simulink model "PandID"  (R2019b)
settings: Solver=VariableStepAuto  StartTime=0.0  StopTime=50  RelTol=1e-3
values from neighbouring files (symbols this model uses):
  L_area = 1    [AFCP_sim.m]
  P_area = 1    [AFCP_sim.m]
  PressureUnit = 1/6894.76    (= 0.000145037680789)    [AFCP_sim.m]
  R_area = 1    [AFCP_sim.m]
  Valve_signal_Unit = 0.00064516    [AFCP_sim.m]
libraries: fl_lib x96, nesl_utility x62, SimscapeFluids_lib x15, simulink x4
(part 2 of 2)

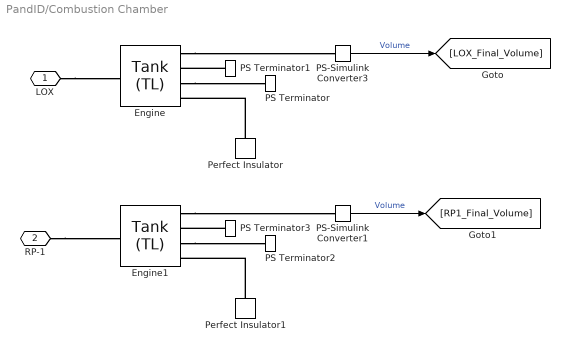
== system PandID/Combustion Chamber ==
  Engine : SimscapeFluids_lib/Thermal Liquid/Tanks & Accumulators/Tank (TL)  pressure_spec=1  tank_pressure=0.101325 MPa  max_capacity=100 m^3  volume_spec=1  tank_area=3 m^2  level_TLU=[0, 3, 5] m  volume_TLU=[0, 4, 6] m^3  inlet_height=0.1 m  inlet_area=0.01 m^2  g=9.81 m/s^2  level_specify=off  level_priority=Low  level=5 m  level_nominal_specify=off  level_nominal_unit=m  level_nominal_value=1  volume_specify=off  volume_priority=Low  volume=5 m^3  volume_nominal_specify=off  volume_nominal_unit=m^3  volume_nominal_value=1  mass_specify=off  mass_priority=Low  mass=5e+3 kg  mass_nominal_specify=off  mass_nominal_unit=kg  mass_nominal_value=1  T_tank_specify=off  T_tank_priority=Low  T_tank=293.15 K  T_tank_nominal_specify=off  T_tank_nominal_unit=K  T_tank_nominal_value=1  inlet_heights_AB=[.1, 0] m  inlet_areas_AB=[L_area, R_area] in^2  inlet_heights_ABC=[.1, .05, 0] m  inlet_areas_ABC=[.01, .01, .01] m^2
      settings: SourceProductName=Simscape Fluids  SourceProductBaseCode=SH  InternalSimscapePortConfiguration="{\"Bottom\":[],\"Left\":[{\"id\":\"A\",\"label\":\"A\",\"type\":\"foundation.thermal_liquid.thermal_liquid\"}],\"Right\":[{\"id\":\"V_out\",\"label\":\"V\",\"type\":\"output\"},{\"id\":\"L_out\",\"label\":\"L\",\"type\":\"output\"},{\"id\":\"T_out\",\"label\":\"T\",\"type\":\"output\"},{\"id\":\"H\",\"label\":\"H\",\"type\":\"foundation.thermal.thermal\"}],\"Top\":[]}"
  Engine1 : SimscapeFluids_lib/Thermal Liquid/Tanks & Accumulators/Tank (TL)  pressure_spec=1  tank_pressure=0.101325 MPa  max_capacity=100 m^3  volume_spec=1  tank_area=3 m^2  level_TLU=[0, 3, 5] m  volume_TLU=[0, 4, 6] m^3  inlet_height=0.1 m  inlet_area=0.01 m^2  g=9.81 m/s^2  level_specify=off  level_priority=Low  level=5 m  level_nominal_specify=off  level_nominal_unit=m  level_nominal_value=1  volume_specify=off  volume_priority=Low  volume=5 m^3  volume_nominal_specify=off  volume_nominal_unit=m^3  volume_nominal_value=1  mass_specify=off  mass_priority=Low  mass=5e+3 kg  mass_nominal_specify=off  mass_nominal_unit=kg  mass_nominal_value=1  T_tank_specify=off  T_tank_priority=Low  T_tank=293.15 K  T_tank_nominal_specify=off  T_tank_nominal_unit=K  T_tank_nominal_value=1  inlet_heights_AB=[.1, 0] m  inlet_areas_AB=[L_area, R_area] in^2  inlet_heights_ABC=[.1, .05, 0] m  inlet_areas_ABC=[.01, .01, .01] m^2
      settings: SourceProductName=Simscape Fluids  SourceProductBaseCode=SH  InternalSimscapePortConfiguration="{\"Bottom\":[],\"Left\":[{\"id\":\"A\",\"label\":\"A\",\"type\":\"foundation.thermal_liquid.thermal_liquid\"}],\"Right\":[{\"id\":\"V_out\",\"label\":\"V\",\"type\":\"output\"},{\"id\":\"L_out\",\"label\":\"L\",\"type\":\"output\"},{\"id\":\"T_out\",\"label\":\"T\",\"type\":\"output\"},{\"id\":\"H\",\"label\":\"H\",\"type\":\"foundation.thermal.thermal\"}],\"Top\":[]}"
  PS Terminator{,1..3} (4 alike) : fl_lib/Physical Signals/Sinks/PS Terminator
      settings: SourceProductName=Simscape
  PS-Simulink Converter1 : nesl_utility/PS-Simulink Converter  PhysicalDomain=network_engine_domain  SubClassName=ps_output  LeftPortType=input  RightPortType=output  PseudoPeriodic=off  Frequencies=[]  Unit=inherit  AffineConversion=off
  PS-Simulink Converter3 : nesl_utility/PS-Simulink Converter  PhysicalDomain=network_engine_domain  SubClassName=ps_output  LeftPortType=input  RightPortType=output  PseudoPeriodic=off  Frequencies=[]  Unit=inherit  AffineConversion=off
  Perfect Insulator : fl_lib/Thermal/Thermal Elements/Perfect Insulator  T_specify=off  T_priority=None  T=0 K  T_nominal_specify=off  T_nominal_unit=K  T_nominal_value=1
      settings: SourceProductName=Simscape
  Perfect Insulator1 : fl_lib/Thermal/Thermal Elements/Perfect Insulator  T_specify=off  T_priority=None  T=0 K  T_nominal_specify=off  T_nominal_unit=K  T_nominal_value=1
      settings: SourceProductName=Simscape
  LOX : PMIOPort  Side=Left
  RP-1 : PMIOPort  Port=2  Side=Left
  wires:
  PS-Simulink Converter3/1 -> [LOX_Final_Volume]  "Volume"
  PS-Simulink Converter1/1 -> [RP1_Final_Volume]  "Volume"
  connections:
  Perfect Insulator/LConn1 -- Engine/RConn4
  Engine/RConn1 -- PS-Simulink Converter3/LConn1
  Engine/RConn3 -- PS Terminator/LConn1
  LOX/RConn1 -- Engine/LConn1
  PS Terminator1/LConn1 -- Engine/RConn2
  RP-1/RConn1 -- Engine1/LConn1
  PS Terminator3/LConn1 -- Engine1/RConn2
  Engine1/RConn3 -- PS Terminator2/LConn1
  Engine1/RConn1 -- PS-Simulink Converter1/LConn1
  Perfect Insulator1/LConn1 -- Engine1/RConn4

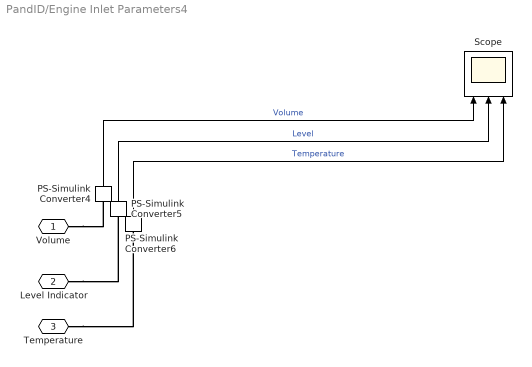
== system PandID/Engine Inlet Parameters4 ==
  PS-Simulink Converter4 : nesl_utility/PS-Simulink Converter  PhysicalDomain=network_engine_domain  SubClassName=ps_output  LeftPortType=input  RightPortType=output  PseudoPeriodic=off  Frequencies=[]  Unit=inherit  AffineConversion=off
  PS-Simulink Converter5 : nesl_utility/PS-Simulink Converter  PhysicalDomain=network_engine_domain  SubClassName=ps_output  LeftPortType=input  RightPortType=output  PseudoPeriodic=off  Frequencies=[]  Unit=inherit  AffineConversion=off
  PS-Simulink Converter6 : nesl_utility/PS-Simulink Converter  PhysicalDomain=network_engine_domain  SubClassName=ps_output  LeftPortType=input  RightPortType=output  PseudoPeriodic=off  Frequencies=[]  Unit=inherit  AffineConversion=off
  Scope : Scope  NumInputPorts=3
  Volume : PMIOPort  Side=Left
  Level Indicator : PMIOPort  Port=2  Side=Left
  Temperature : PMIOPort  Port=3  Side=Left
  wires:
  PS-Simulink Converter6/1 -> Scope/3  "Temperature"
  PS-Simulink Converter4/1 -> Scope/1  "Volume"
  PS-Simulink Converter5/1 -> Scope/2  "Level"
  connections:
  Temperature/RConn1 -- PS-Simulink Converter6/LConn1
  Volume/RConn1 -- PS-Simulink Converter4/LConn1
  Level Indicator/RConn1 -- PS-Simulink Converter5/LConn1

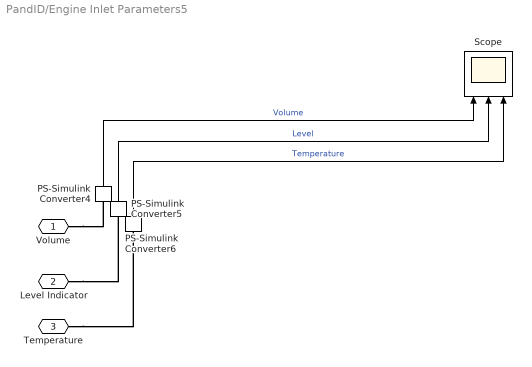
== system PandID/Engine Inlet Parameters5 ==
  PS-Simulink Converter4 : nesl_utility/PS-Simulink Converter  PhysicalDomain=network_engine_domain  SubClassName=ps_output  LeftPortType=input  RightPortType=output  PseudoPeriodic=off  Frequencies=[]  Unit=inherit  AffineConversion=off
  PS-Simulink Converter5 : nesl_utility/PS-Simulink Converter  PhysicalDomain=network_engine_domain  SubClassName=ps_output  LeftPortType=input  RightPortType=output  PseudoPeriodic=off  Frequencies=[]  Unit=inherit  AffineConversion=off
  PS-Simulink Converter6 : nesl_utility/PS-Simulink Converter  PhysicalDomain=network_engine_domain  SubClassName=ps_output  LeftPortType=input  RightPortType=output  PseudoPeriodic=off  Frequencies=[]  Unit=inherit  AffineConversion=off
  Scope : Scope  NumInputPorts=3
  Volume : PMIOPort  Side=Left
  Level Indicator : PMIOPort  Port=2  Side=Left
  Temperature : PMIOPort  Port=3  Side=Left
  wires:
  PS-Simulink Converter5/1 -> Scope/2  "Level"
  PS-Simulink Converter4/1 -> Scope/1  "Volume"
  PS-Simulink Converter6/1 -> Scope/3  "Temperature"
  connections:
  Level Indicator/RConn1 -- PS-Simulink Converter5/LConn1
  Volume/RConn1 -- PS-Simulink Converter4/LConn1
  Temperature/RConn1 -- PS-Simulink Converter6/LConn1

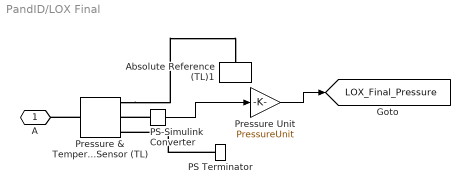
== system PandID/LOX Final ==
  Absolute Reference (TL)1 : fl_lib/Thermal Liquid/Elements/Absolute Reference (TL)
      settings: SourceProductName=Simscape  SourceProductBaseCode=SS
  PS Terminator : fl_lib/Physical Signals/Sinks/PS Terminator
      settings: SourceProductName=Simscape
  PS-Simulink Converter : nesl_utility/PS-Simulink Converter  PhysicalDomain=network_engine_domain  SubClassName=ps_output  LeftPortType=input  RightPortType=output  PseudoPeriodic=off  Frequencies=[]  Unit=inherit  AffineConversion=off
  Pressure & Temperature Sensor (TL) : fl_lib/Thermal Liquid/Sensors/Pressure & Temperature Sensor (TL)
      settings: SourceProductName=Simscape  SourceProductBaseCode=SS  InternalSimscapePortConfiguration="{\"Bottom\":[],\"Left\":[{\"id\":\"A\",\"label\":\"A\",\"type\":\"foundation.thermal_liquid.thermal_liquid\"}],\"Right\":[{\"id\":\"B\",\"label\":\"B\",\"type\":\"foundation.thermal_liquid.thermal_liquid\"},{\"id\":\"P\",\"label\":\"P\",\"type\":\"output\"},{\"id\":\"T\",\"label\":\"T\",\"type\":\"output\"}],\"Top\":[]}"
  Pressure Unit : Gain  Gain=PressureUnit
  A : PMIOPort  Side=Left
  tag scope: LOX_Final_Pressure=global
  wires:
  Pressure Unit/1 -> [LOX_Final_Pressure]
  PS-Simulink Converter/1 -> Pressure Unit/1
  connections:
  PS Terminator/LConn1 -- Pressure & Temperature Sensor (TL)/RConn3
  PS-Simulink Converter/LConn1 -- Pressure & Temperature Sensor (TL)/RConn2
  Pressure & Temperature Sensor (TL)/LConn1 -- A/RConn1
  Pressure & Temperature Sensor (TL)/RConn1 -- Absolute Reference (TL)1/LConn1

== system PandID/LOX Tank ==
  Controlled Pressure Source (TL) : fl_lib/Thermal Liquid/Sources/Controlled Pressure Source (TL)  area=0.01 in^2
      settings: SourceProductName=Simscape  SourceProductBaseCode=SS  InternalSimscapePortConfiguration="{\"Bottom\":[],\"Left\":[{\"id\":\"A\",\"label\":\"A\",\"type\":\"foundation.thermal_liquid.thermal_liquid\"},{\"id\":\"P\",\"label\":\"P\",\"type\":\"input\"}],\"Right\":[{\"id\":\"B\",\"label\":\"B\",\"type\":\"foundation.thermal_liquid.thermal_liquid\"}],\"Top\":[]}"
  Reservoir (TL) : fl_lib/Thermal Liquid/Elements/Reservoir (TL)  pressure_spec=foundation.enum.pressure_spec.atmospheric  reservoir_pressure=0.101325 MPa  reservoir_temperature=293.15 K  area=L_area in^2
      settings: SourceProductName=Simscape  SourceProductBaseCode=SS
  LOX : PMIOPort  Side=Right
  Pressurant input : PMIOPort  Port=2  Side=Left
  connections:
  Reservoir (TL)/LConn1 -- Controlled Pressure Source (TL)/LConn1
  Controlled Pressure Source (TL)/LConn2 -- Pressurant input/RConn1
  Controlled Pressure Source (TL)/RConn1 -- LOX/RConn1

== system PandID/Pressurant Tank ==
  Pressure Source (TL) : fl_lib/Thermal Liquid/Sources/Pressure Source (TL)  commanded_pressure=Pressurant_tank_initial_pressure psi  area=P_area in^2
      settings: SourceProductName=Simscape  SourceProductBaseCode=SS  InternalSimscapePortConfiguration="{\"Bottom\":[],\"Left\":[{\"id\":\"A\",\"label\":\"A\",\"type\":\"foundation.thermal_liquid.thermal_liquid\"}],\"Right\":[{\"id\":\"B\",\"label\":\"B\",\"type\":\"foundation.thermal_liquid.thermal_liquid\"}],\"Top\":[]}"
  Reservoir (TL) : fl_lib/Thermal Liquid/Elements/Reservoir (TL)  pressure_spec=foundation.enum.pressure_spec.atmospheric  reservoir_pressure=0.101325 MPa  reservoir_temperature=293.15 K  area=1 in^2
      settings: SourceProductName=Simscape  SourceProductBaseCode=SS
  LOX : PMIOPort  Side=Right
  connections:
  Reservoir (TL)/LConn1 -- Pressure Source (TL)/LConn1
  Pressure Source (TL)/RConn1 -- LOX/RConn1

== system PandID/Pressurant Tank1 ==
  Pressure Source (TL) : fl_lib/Thermal Liquid/Sources/Pressure Source (TL)  commanded_pressure=Pressurant_tank_initial_pressure psi  area=P_area in^2
      settings: SourceProductName=Simscape  SourceProductBaseCode=SS  InternalSimscapePortConfiguration="{\"Bottom\":[],\"Left\":[{\"id\":\"A\",\"label\":\"A\",\"type\":\"foundation.thermal_liquid.thermal_liquid\"}],\"Right\":[{\"id\":\"B\",\"label\":\"B\",\"type\":\"foundation.thermal_liquid.thermal_liquid\"}],\"Top\":[]}"
  Reservoir (TL) : fl_lib/Thermal Liquid/Elements/Reservoir (TL)  pressure_spec=foundation.enum.pressure_spec.atmospheric  reservoir_pressure=0.101325 MPa  reservoir_temperature=293.15 K  area=1 in^2
      settings: SourceProductName=Simscape  SourceProductBaseCode=SS
  LOX : PMIOPort  Side=Right
  connections:
  Pressure Source (TL)/RConn1 -- LOX/RConn1
  Reservoir (TL)/LConn1 -- Pressure Source (TL)/LConn1

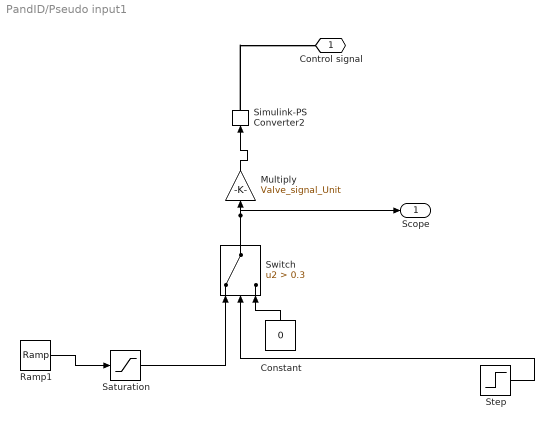
== system PandID/Pseudo input1 ==
  Constant : Constant  Value=0
  Multiply : Gain  Gain=Valve_signal_Unit
  Ramp1 : simulink/Sources/Ramp  slope=0.05  start=100  InitialOutput=0
  Saturation : Saturate  UpperLimit=P_area  LowerLimit=0
  Simulink-PS Converter2 : nesl_utility/Simulink-PS Converter  PhysicalDomain=network_engine_domain  SubClassName=ps_input  LeftPortType=input  RightPortType=output  PseudoPeriodic=off  Frequencies=[]  NoiseDistribution=none  NoiseParameters=[]  Unit=m^2  AffineConversion=off  FilteringAndDerivatives=provide  SimscapeFilterOrder=1  InputFilterTimeConstant=0.001  UdotUserProvided=0
  Step : Step  Time=500  Before=1  After=0  SampleTime=0
  Switch : Switch  Criteria=u2 > Threshold  Threshold=0.3
  Control signal : PMIOPort  Side=Right
  Scope : Outport
  wires:
  Switch/1 -> Scope/1, Multiply/1
  Constant/1 -> Switch/3
  Step/1 -> Switch/2
  Ramp1/1 -> Saturation/1
  Saturation/1 -> Switch/1
  Multiply/1 -> Simulink-PS Converter2/1
  connections:
  Simulink-PS Converter2/RConn1 -- Control signal/RConn1

== system PandID/Pseudo input2 ==
  Constant : Constant  Value=0
  Ramp1 : simulink/Sources/Ramp  slope=0.0005  start=20  InitialOutput=0
  Simulink-PS Converter2 : nesl_utility/Simulink-PS Converter  PhysicalDomain=network_engine_domain  SubClassName=ps_input  LeftPortType=input  RightPortType=output  PseudoPeriodic=off  Frequencies=[]  NoiseDistribution=none  NoiseParameters=[]  Unit=m^2  AffineConversion=off  FilteringAndDerivatives=provide  SimscapeFilterOrder=1  InputFilterTimeConstant=0.001  UdotUserProvided=0
  Step : Step  Time=200  Before=1  After=0  SampleTime=0
  Switch : Switch  Criteria=u2 > Threshold  Threshold=0.3
  Control signal : PMIOPort  Side=Right
  Scope : Outport
  wires:
  Ramp1/1 -> Switch/1
  Step/1 -> Switch/2
  Constant/1 -> Switch/3
  Switch/1 -> Simulink-PS Converter2/1, Scope/1
  connections:
  Simulink-PS Converter2/RConn1 -- Control signal/RConn1

== system PandID/Pseudo input3 ==
  Constant : Constant  Value=0
  Ramp1 : simulink/Sources/Ramp  slope=0.0005  start=20  InitialOutput=0
  Simulink-PS Converter2 : nesl_utility/Simulink-PS Converter  PhysicalDomain=network_engine_domain  SubClassName=ps_input  LeftPortType=input  RightPortType=output  PseudoPeriodic=off  Frequencies=[]  NoiseDistribution=none  NoiseParameters=[]  Unit=m^2  AffineConversion=off  FilteringAndDerivatives=provide  SimscapeFilterOrder=1  InputFilterTimeConstant=0.001  UdotUserProvided=0
  Step : Step  Time=200  Before=1  After=0  SampleTime=0
  Switch : Switch  Criteria=u2 > Threshold  Threshold=0.3
  Control signal : PMIOPort  Side=Right
  Scope : Outport
  wires:
  Ramp1/1 -> Switch/1
  Step/1 -> Switch/2
  Constant/1 -> Switch/3
  Switch/1 -> Simulink-PS Converter2/1, Scope/1
  connections:
  Simulink-PS Converter2/RConn1 -- Control signal/RConn1

== system PandID/RP-1 Tank ==
  Controlled Pressure Source (TL) : fl_lib/Thermal Liquid/Sources/Controlled Pressure Source (TL)  area=R_area in^2
      settings: SourceProductName=Simscape  SourceProductBaseCode=SS  InternalSimscapePortConfiguration="{\"Bottom\":[],\"Left\":[{\"id\":\"A\",\"label\":\"A\",\"type\":\"foundation.thermal_liquid.thermal_liquid\"},{\"id\":\"P\",\"label\":\"P\",\"type\":\"input\"}],\"Right\":[{\"id\":\"B\",\"label\":\"B\",\"type\":\"foundation.thermal_liquid.thermal_liquid\"}],\"Top\":[]}"
  Reservoir (TL) : fl_lib/Thermal Liquid/Elements/Reservoir (TL)  pressure_spec=foundation.enum.pressure_spec.atmospheric  reservoir_pressure=0.101325 MPa  reservoir_temperature=293.15 K  area=R_area in^2
      settings: SourceProductName=Simscape  SourceProductBaseCode=SS
  LOX : PMIOPort  Side=Right
  Pressurant input : PMIOPort  Port=2  Side=Left
  connections:
  Controlled Pressure Source (TL)/RConn1 -- LOX/RConn1
  Controlled Pressure Source (TL)/LConn2 -- Pressurant input/RConn1
  Reservoir (TL)/LConn1 -- Controlled Pressure Source (TL)/LConn1

== system PandID/RP1 Final ==
  Absolute Reference (TL)1 : fl_lib/Thermal Liquid/Elements/Absolute Reference (TL)
      settings: SourceProductName=Simscape  SourceProductBaseCode=SS
  PS Terminator : fl_lib/Physical Signals/Sinks/PS Terminator
      settings: SourceProductName=Simscape
  PS-Simulink Converter : nesl_utility/PS-Simulink Converter  PhysicalDomain=network_engine_domain  SubClassName=ps_output  LeftPortType=input  RightPortType=output  PseudoPeriodic=off  Frequencies=[]  Unit=inherit  AffineConversion=off
  Pressure & Temperature Sensor (TL) : fl_lib/Thermal Liquid/Sensors/Pressure & Temperature Sensor (TL)
      settings: SourceProductName=Simscape  SourceProductBaseCode=SS  InternalSimscapePortConfiguration="{\"Bottom\":[],\"Left\":[{\"id\":\"A\",\"label\":\"A\",\"type\":\"foundation.thermal_liquid.thermal_liquid\"}],\"Right\":[{\"id\":\"B\",\"label\":\"B\",\"type\":\"foundation.thermal_liquid.thermal_liquid\"},{\"id\":\"P\",\"label\":\"P\",\"type\":\"output\"},{\"id\":\"T\",\"label\":\"T\",\"type\":\"output\"}],\"Top\":[]}"
  Pressure Unit : Gain  Gain=PressureUnit
  A : PMIOPort  Side=Left
  tag scope: RP1_Final_Pressure=global
  wires:
  PS-Simulink Converter/1 -> Pressure Unit/1
  Pressure Unit/1 -> [RP1_Final_Pressure]
  connections:
  Pressure & Temperature Sensor (TL)/RConn1 -- Absolute Reference (TL)1/LConn1
  Pressure & Temperature Sensor (TL)/LConn1 -- A/RConn1
  PS-Simulink Converter/LConn1 -- Pressure & Temperature Sensor (TL)/RConn2
  PS Terminator/LConn1 -- Pressure & Temperature Sensor (TL)/RConn3

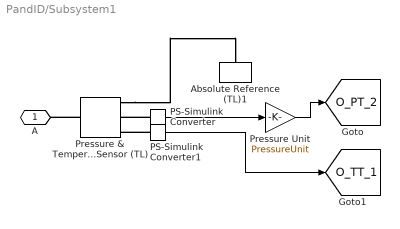
== system PandID/Subsystem1 ==
  Absolute Reference (TL)1 : fl_lib/Thermal Liquid/Elements/Absolute Reference (TL)
      settings: SourceProductName=Simscape  SourceProductBaseCode=SS
  PS-Simulink Converter : nesl_utility/PS-Simulink Converter  PhysicalDomain=network_engine_domain  SubClassName=ps_output  LeftPortType=input  RightPortType=output  PseudoPeriodic=off  Frequencies=[]  Unit=inherit  AffineConversion=off
  PS-Simulink Converter1 : nesl_utility/PS-Simulink Converter  PhysicalDomain=network_engine_domain  SubClassName=ps_output  LeftPortType=input  RightPortType=output  PseudoPeriodic=off  Frequencies=[]  Unit=inherit  AffineConversion=off
  Pressure & Temperature Sensor (TL) : fl_lib/Thermal Liquid/Sensors/Pressure & Temperature Sensor (TL)
      settings: SourceProductName=Simscape  SourceProductBaseCode=SS  InternalSimscapePortConfiguration="{\"Bottom\":[],\"Left\":[{\"id\":\"A\",\"label\":\"A\",\"type\":\"foundation.thermal_liquid.thermal_liquid\"}],\"Right\":[{\"id\":\"B\",\"label\":\"B\",\"type\":\"foundation.thermal_liquid.thermal_liquid\"},{\"id\":\"P\",\"label\":\"P\",\"type\":\"output\"},{\"id\":\"T\",\"label\":\"T\",\"type\":\"output\"}],\"Top\":[]}"
  Pressure Unit : Gain  Gain=PressureUnit
  A : PMIOPort  Side=Left
  tag scope: O_PT_2=global, O_TT_1=global
  wires:
  PS-Simulink Converter/1 -> Pressure Unit/1
  PS-Simulink Converter1/1 -> [O_TT_1]
  Pressure Unit/1 -> [O_PT_2]
  connections:
  Pressure & Temperature Sensor (TL)/RConn1 -- Absolute Reference (TL)1/LConn1
  Pressure & Temperature Sensor (TL)/LConn1 -- A/RConn1
  PS-Simulink Converter/LConn1 -- Pressure & Temperature Sensor (TL)/RConn2
  PS-Simulink Converter1/LConn1 -- Pressure & Temperature Sensor (TL)/RConn3

== system PandID/Subsystem10 ==
  Absolute Reference (TL)1 : fl_lib/Thermal Liquid/Elements/Absolute Reference (TL)
      settings: SourceProductName=Simscape  SourceProductBaseCode=SS
  PS Terminator : fl_lib/Physical Signals/Sinks/PS Terminator
      settings: SourceProductName=Simscape
  Pressure & Temperature Sensor (TL) : fl_lib/Thermal Liquid/Sensors/Pressure & Temperature Sensor (TL)
      settings: SourceProductName=Simscape  SourceProductBaseCode=SS  InternalSimscapePortConfiguration="{\"Bottom\":[],\"Left\":[{\"id\":\"A\",\"label\":\"A\",\"type\":\"foundation.thermal_liquid.thermal_liquid\"}],\"Right\":[{\"id\":\"B\",\"label\":\"B\",\"type\":\"foundation.thermal_liquid.thermal_liquid\"},{\"id\":\"P\",\"label\":\"P\",\"type\":\"output\"},{\"id\":\"T\",\"label\":\"T\",\"type\":\"output\"}],\"Top\":[]}"
  A : PMIOPort  Side=Left
  LOX : PMIOPort  Port=2  Side=Right
  connections:
  PS Terminator/LConn1 -- Pressure & Temperature Sensor (TL)/RConn3
  Pressure & Temperature Sensor (TL)/RConn2 -- LOX/RConn1
  Pressure & Temperature Sensor (TL)/LConn1 -- A/RConn1
  Pressure & Temperature Sensor (TL)/RConn1 -- Absolute Reference (TL)1/LConn1

== system PandID/Subsystem2 ==
  Absolute Reference (TL)1 : fl_lib/Thermal Liquid/Elements/Absolute Reference (TL)
      settings: SourceProductName=Simscape  SourceProductBaseCode=SS
  PS Terminator : fl_lib/Physical Signals/Sinks/PS Terminator
      settings: SourceProductName=Simscape
  PS-Simulink Converter : nesl_utility/PS-Simulink Converter  PhysicalDomain=network_engine_domain  SubClassName=ps_output  LeftPortType=input  RightPortType=output  PseudoPeriodic=off  Frequencies=[]  Unit=inherit  AffineConversion=off
  Pressure & Temperature Sensor (TL) : fl_lib/Thermal Liquid/Sensors/Pressure & Temperature Sensor (TL)
      settings: SourceProductName=Simscape  SourceProductBaseCode=SS  InternalSimscapePortConfiguration="{\"Bottom\":[],\"Left\":[{\"id\":\"A\",\"label\":\"A\",\"type\":\"foundation.thermal_liquid.thermal_liquid\"}],\"Right\":[{\"id\":\"B\",\"label\":\"B\",\"type\":\"foundation.thermal_liquid.thermal_liquid\"},{\"id\":\"P\",\"label\":\"P\",\"type\":\"output\"},{\"id\":\"T\",\"label\":\"T\",\"type\":\"output\"}],\"Top\":[]}"
  Pressure Unit : Gain  Gain=PressureUnit
  A : PMIOPort  Side=Left
  tag scope: O_PT_3=global
  wires:
  PS-Simulink Converter/1 -> Pressure Unit/1
  Pressure Unit/1 -> [O_PT_3]
  connections:
  PS Terminator/LConn1 -- Pressure & Temperature Sensor (TL)/RConn3
  PS-Simulink Converter/LConn1 -- Pressure & Temperature Sensor (TL)/RConn2
  Pressure & Temperature Sensor (TL)/LConn1 -- A/RConn1
  Pressure & Temperature Sensor (TL)/RConn1 -- Absolute Reference (TL)1/LConn1

== system PandID/Subsystem3 ==
  Absolute Reference (TL)1 : fl_lib/Thermal Liquid/Elements/Absolute Reference (TL)
      settings: SourceProductName=Simscape  SourceProductBaseCode=SS
  PS Terminator : fl_lib/Physical Signals/Sinks/PS Terminator
      settings: SourceProductName=Simscape
  PS-Simulink Converter : nesl_utility/PS-Simulink Converter  PhysicalDomain=network_engine_domain  SubClassName=ps_output  LeftPortType=input  RightPortType=output  PseudoPeriodic=off  Frequencies=[]  Unit=inherit  AffineConversion=off
  Pressure & Temperature Sensor (TL) : fl_lib/Thermal Liquid/Sensors/Pressure & Temperature Sensor (TL)
      settings: SourceProductName=Simscape  SourceProductBaseCode=SS  InternalSimscapePortConfiguration="{\"Bottom\":[],\"Left\":[{\"id\":\"A\",\"label\":\"A\",\"type\":\"foundation.thermal_liquid.thermal_liquid\"}],\"Right\":[{\"id\":\"B\",\"label\":\"B\",\"type\":\"foundation.thermal_liquid.thermal_liquid\"},{\"id\":\"P\",\"label\":\"P\",\"type\":\"output\"},{\"id\":\"T\",\"label\":\"T\",\"type\":\"output\"}],\"Top\":[]}"
  Pressure Unit : Gain  Gain=PressureUnit
  A : PMIOPort  Side=Left
  tag scope: O_PT_1=global
  wires:
  PS-Simulink Converter/1 -> Pressure Unit/1
  Pressure Unit/1 -> [O_PT_1]
  connections:
  PS Terminator/LConn1 -- Pressure & Temperature Sensor (TL)/RConn3
  PS-Simulink Converter/LConn1 -- Pressure & Temperature Sensor (TL)/RConn2
  Pressure & Temperature Sensor (TL)/LConn1 -- A/RConn1
  Pressure & Temperature Sensor (TL)/RConn1 -- Absolute Reference (TL)1/LConn1

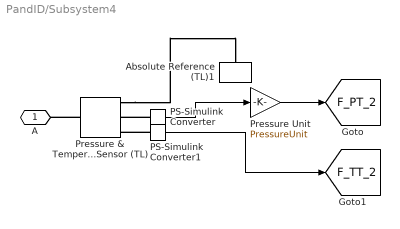
== system PandID/Subsystem4 ==
  Absolute Reference (TL)1 : fl_lib/Thermal Liquid/Elements/Absolute Reference (TL)
      settings: SourceProductName=Simscape  SourceProductBaseCode=SS
  PS-Simulink Converter : nesl_utility/PS-Simulink Converter  PhysicalDomain=network_engine_domain  SubClassName=ps_output  LeftPortType=input  RightPortType=output  PseudoPeriodic=off  Frequencies=[]  Unit=inherit  AffineConversion=off
  PS-Simulink Converter1 : nesl_utility/PS-Simulink Converter  PhysicalDomain=network_engine_domain  SubClassName=ps_output  LeftPortType=input  RightPortType=output  PseudoPeriodic=off  Frequencies=[]  Unit=inherit  AffineConversion=off
  Pressure & Temperature Sensor (TL) : fl_lib/Thermal Liquid/Sensors/Pressure & Temperature Sensor (TL)
      settings: SourceProductName=Simscape  SourceProductBaseCode=SS  InternalSimscapePortConfiguration="{\"Bottom\":[],\"Left\":[{\"id\":\"A\",\"label\":\"A\",\"type\":\"foundation.thermal_liquid.thermal_liquid\"}],\"Right\":[{\"id\":\"B\",\"label\":\"B\",\"type\":\"foundation.thermal_liquid.thermal_liquid\"},{\"id\":\"P\",\"label\":\"P\",\"type\":\"output\"},{\"id\":\"T\",\"label\":\"T\",\"type\":\"output\"}],\"Top\":[]}"
  Pressure Unit : Gain  Gain=PressureUnit
  A : PMIOPort  Side=Left
  tag scope: F_PT_2=global, F_TT_2=global
  wires:
  PS-Simulink Converter1/1 -> [F_TT_2]
  PS-Simulink Converter/1 -> Pressure Unit/1
  Pressure Unit/1 -> [F_PT_2]
  connections:
  PS-Simulink Converter1/LConn1 -- Pressure & Temperature Sensor (TL)/RConn3
  PS-Simulink Converter/LConn1 -- Pressure & Temperature Sensor (TL)/RConn2
  Pressure & Temperature Sensor (TL)/LConn1 -- A/RConn1
  Pressure & Temperature Sensor (TL)/RConn1 -- Absolute Reference (TL)1/LConn1

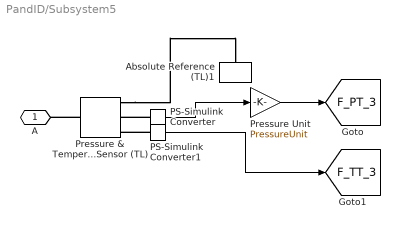
== system PandID/Subsystem5 ==
  Absolute Reference (TL)1 : fl_lib/Thermal Liquid/Elements/Absolute Reference (TL)
      settings: SourceProductName=Simscape  SourceProductBaseCode=SS
  PS-Simulink Converter : nesl_utility/PS-Simulink Converter  PhysicalDomain=network_engine_domain  SubClassName=ps_output  LeftPortType=input  RightPortType=output  PseudoPeriodic=off  Frequencies=[]  Unit=inherit  AffineConversion=off
  PS-Simulink Converter1 : nesl_utility/PS-Simulink Converter  PhysicalDomain=network_engine_domain  SubClassName=ps_output  LeftPortType=input  RightPortType=output  PseudoPeriodic=off  Frequencies=[]  Unit=inherit  AffineConversion=off
  Pressure & Temperature Sensor (TL) : fl_lib/Thermal Liquid/Sensors/Pressure & Temperature Sensor (TL)
      settings: SourceProductName=Simscape  SourceProductBaseCode=SS  InternalSimscapePortConfiguration="{\"Bottom\":[],\"Left\":[{\"id\":\"A\",\"label\":\"A\",\"type\":\"foundation.thermal_liquid.thermal_liquid\"}],\"Right\":[{\"id\":\"B\",\"label\":\"B\",\"type\":\"foundation.thermal_liquid.thermal_liquid\"},{\"id\":\"P\",\"label\":\"P\",\"type\":\"output\"},{\"id\":\"T\",\"label\":\"T\",\"type\":\"output\"}],\"Top\":[]}"
  Pressure Unit : Gain  Gain=PressureUnit
  A : PMIOPort  Side=Left
  tag scope: F_PT_3=global, F_TT_3=global
  wires:
  PS-Simulink Converter/1 -> Pressure Unit/1
  PS-Simulink Converter1/1 -> [F_TT_3]
  Pressure Unit/1 -> [F_PT_3]
  connections:
  Pressure & Temperature Sensor (TL)/RConn1 -- Absolute Reference (TL)1/LConn1
  Pressure & Temperature Sensor (TL)/LConn1 -- A/RConn1
  PS-Simulink Converter/LConn1 -- Pressure & Temperature Sensor (TL)/RConn2
  PS-Simulink Converter1/LConn1 -- Pressure & Temperature Sensor (TL)/RConn3

== system PandID/Subsystem6 ==
  Absolute Reference (TL)1 : fl_lib/Thermal Liquid/Elements/Absolute Reference (TL)
      settings: SourceProductName=Simscape  SourceProductBaseCode=SS
  PS Terminator : fl_lib/Physical Signals/Sinks/PS Terminator
      settings: SourceProductName=Simscape
  PS-Simulink Converter : nesl_utility/PS-Simulink Converter  PhysicalDomain=network_engine_domain  SubClassName=ps_output  LeftPortType=input  RightPortType=output  PseudoPeriodic=off  Frequencies=[]  Unit=inherit  AffineConversion=off
  Pressure & Temperature Sensor (TL) : fl_lib/Thermal Liquid/Sensors/Pressure & Temperature Sensor (TL)
      settings: SourceProductName=Simscape  SourceProductBaseCode=SS  InternalSimscapePortConfiguration="{\"Bottom\":[],\"Left\":[{\"id\":\"A\",\"label\":\"A\",\"type\":\"foundation.thermal_liquid.thermal_liquid\"}],\"Right\":[{\"id\":\"B\",\"label\":\"B\",\"type\":\"foundation.thermal_liquid.thermal_liquid\"},{\"id\":\"P\",\"label\":\"P\",\"type\":\"output\"},{\"id\":\"T\",\"label\":\"T\",\"type\":\"output\"}],\"Top\":[]}"
  Pressure Unit : Gain  Gain=PressureUnit
  A : PMIOPort  Side=Left
  tag scope: F_PT_1=global
  wires:
  PS-Simulink Converter/1 -> Pressure Unit/1
  Pressure Unit/1 -> [F_PT_1]
  connections:
  Pressure & Temperature Sensor (TL)/RConn1 -- Absolute Reference (TL)1/LConn1
  Pressure & Temperature Sensor (TL)/LConn1 -- A/RConn1
  PS-Simulink Converter/LConn1 -- Pressure & Temperature Sensor (TL)/RConn2
  PS Terminator/LConn1 -- Pressure & Temperature Sensor (TL)/RConn3

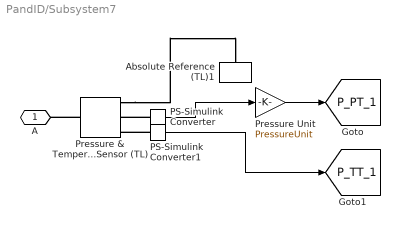
== system PandID/Subsystem7 ==
  Absolute Reference (TL)1 : fl_lib/Thermal Liquid/Elements/Absolute Reference (TL)
      settings: SourceProductName=Simscape  SourceProductBaseCode=SS
  PS-Simulink Converter : nesl_utility/PS-Simulink Converter  PhysicalDomain=network_engine_domain  SubClassName=ps_output  LeftPortType=input  RightPortType=output  PseudoPeriodic=off  Frequencies=[]  Unit=inherit  AffineConversion=off
  PS-Simulink Converter1 : nesl_utility/PS-Simulink Converter  PhysicalDomain=network_engine_domain  SubClassName=ps_output  LeftPortType=input  RightPortType=output  PseudoPeriodic=off  Frequencies=[]  Unit=inherit  AffineConversion=off
  Pressure & Temperature Sensor (TL) : fl_lib/Thermal Liquid/Sensors/Pressure & Temperature Sensor (TL)
      settings: SourceProductName=Simscape  SourceProductBaseCode=SS  InternalSimscapePortConfiguration="{\"Bottom\":[],\"Left\":[{\"id\":\"A\",\"label\":\"A\",\"type\":\"foundation.thermal_liquid.thermal_liquid\"}],\"Right\":[{\"id\":\"B\",\"label\":\"B\",\"type\":\"foundation.thermal_liquid.thermal_liquid\"},{\"id\":\"P\",\"label\":\"P\",\"type\":\"output\"},{\"id\":\"T\",\"label\":\"T\",\"type\":\"output\"}],\"Top\":[]}"
  Pressure Unit : Gain  Gain=PressureUnit
  A : PMIOPort  Side=Left
  tag scope: P_PT_1=global, P_TT_1=global
  wires:
  PS-Simulink Converter/1 -> Pressure Unit/1
  PS-Simulink Converter1/1 -> [P_TT_1]
  Pressure Unit/1 -> [P_PT_1]
  connections:
  Pressure & Temperature Sensor (TL)/RConn1 -- Absolute Reference (TL)1/LConn1
  Pressure & Temperature Sensor (TL)/LConn1 -- A/RConn1
  PS-Simulink Converter/LConn1 -- Pressure & Temperature Sensor (TL)/RConn2
  PS-Simulink Converter1/LConn1 -- Pressure & Temperature Sensor (TL)/RConn3

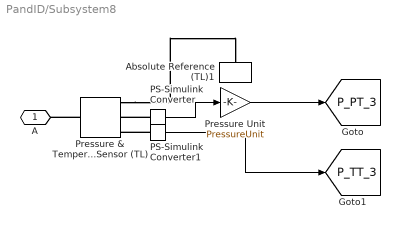
== system PandID/Subsystem8 ==
  Absolute Reference (TL)1 : fl_lib/Thermal Liquid/Elements/Absolute Reference (TL)
      settings: SourceProductName=Simscape  SourceProductBaseCode=SS
  PS-Simulink Converter : nesl_utility/PS-Simulink Converter  PhysicalDomain=network_engine_domain  SubClassName=ps_output  LeftPortType=input  RightPortType=output  PseudoPeriodic=off  Frequencies=[]  Unit=inherit  AffineConversion=off
  PS-Simulink Converter1 : nesl_utility/PS-Simulink Converter  PhysicalDomain=network_engine_domain  SubClassName=ps_output  LeftPortType=input  RightPortType=output  PseudoPeriodic=off  Frequencies=[]  Unit=inherit  AffineConversion=off
  Pressure & Temperature Sensor (TL) : fl_lib/Thermal Liquid/Sensors/Pressure & Temperature Sensor (TL)
      settings: SourceProductName=Simscape  SourceProductBaseCode=SS  InternalSimscapePortConfiguration="{\"Bottom\":[],\"Left\":[{\"id\":\"A\",\"label\":\"A\",\"type\":\"foundation.thermal_liquid.thermal_liquid\"}],\"Right\":[{\"id\":\"B\",\"label\":\"B\",\"type\":\"foundation.thermal_liquid.thermal_liquid\"},{\"id\":\"P\",\"label\":\"P\",\"type\":\"output\"},{\"id\":\"T\",\"label\":\"T\",\"type\":\"output\"}],\"Top\":[]}"
  Pressure Unit : Gain  Gain=PressureUnit
  A : PMIOPort  Side=Left
  tag scope: P_PT_3=global, P_TT_3=global
  wires:
  PS-Simulink Converter1/1 -> [P_TT_3]
  PS-Simulink Converter/1 -> Pressure Unit/1
  Pressure Unit/1 -> [P_PT_3]
  connections:
  PS-Simulink Converter1/LConn1 -- Pressure & Temperature Sensor (TL)/RConn3
  PS-Simulink Converter/LConn1 -- Pressure & Temperature Sensor (TL)/RConn2
  Pressure & Temperature Sensor (TL)/LConn1 -- A/RConn1
  Pressure & Temperature Sensor (TL)/RConn1 -- Absolute Reference (TL)1/LConn1

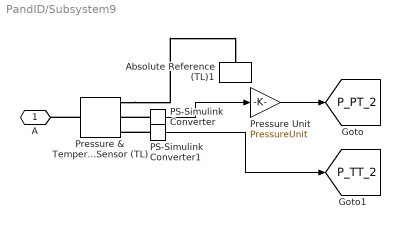
== system PandID/Subsystem9 ==
  Absolute Reference (TL)1 : fl_lib/Thermal Liquid/Elements/Absolute Reference (TL)
      settings: SourceProductName=Simscape  SourceProductBaseCode=SS
  PS-Simulink Converter : nesl_utility/PS-Simulink Converter  PhysicalDomain=network_engine_domain  SubClassName=ps_output  LeftPortType=input  RightPortType=output  PseudoPeriodic=off  Frequencies=[]  Unit=inherit  AffineConversion=off
  PS-Simulink Converter1 : nesl_utility/PS-Simulink Converter  PhysicalDomain=network_engine_domain  SubClassName=ps_output  LeftPortType=input  RightPortType=output  PseudoPeriodic=off  Frequencies=[]  Unit=inherit  AffineConversion=off
  Pressure & Temperature Sensor (TL) : fl_lib/Thermal Liquid/Sensors/Pressure & Temperature Sensor (TL)
      settings: SourceProductName=Simscape  SourceProductBaseCode=SS  InternalSimscapePortConfiguration="{\"Bottom\":[],\"Left\":[{\"id\":\"A\",\"label\":\"A\",\"type\":\"foundation.thermal_liquid.thermal_liquid\"}],\"Right\":[{\"id\":\"B\",\"label\":\"B\",\"type\":\"foundation.thermal_liquid.thermal_liquid\"},{\"id\":\"P\",\"label\":\"P\",\"type\":\"output\"},{\"id\":\"T\",\"label\":\"T\",\"type\":\"output\"}],\"Top\":[]}"
  Pressure Unit : Gain  Gain=PressureUnit
  A : PMIOPort  Side=Left
  tag scope: P_PT_2=global, P_TT_2=global
  wires:
  PS-Simulink Converter/1 -> Pressure Unit/1
  PS-Simulink Converter1/1 -> [P_TT_2]
  Pressure Unit/1 -> [P_PT_2]
  connections:
  Pressure & Temperature Sensor (TL)/RConn1 -- Absolute Reference (TL)1/LConn1
  Pressure & Temperature Sensor (TL)/LConn1 -- A/RConn1
  PS-Simulink Converter/LConn1 -- Pressure & Temperature Sensor (TL)/RConn2
  PS-Simulink Converter1/LConn1 -- Pressure & Temperature Sensor (TL)/RConn3

== system PandID/Valve Actuation Block ==
  Boolean signal : Inport
  Constant : Constant  Value=0
  Constant1 : Constant  Value=P_area
  Multiply : Gain  Gain=Valve_signal_Unit
  Simulink-PS Converter2 : nesl_utility/Simulink-PS Converter  PhysicalDomain=network_engine_domain  SubClassName=ps_input  LeftPortType=input  RightPortType=output  PseudoPeriodic=off  Frequencies=[]  NoiseDistribution=none  NoiseParameters=[]  Unit=m^2  AffineConversion=off  FilteringAndDerivatives=provide  SimscapeFilterOrder=1  InputFilterTimeConstant=0.001  UdotUserProvided=0
  Switch : Switch  Threshold=1
  Control signal : PMIOPort  Side=Right
  wires:
  Multiply/1 -> Simulink-PS Converter2/1
  Switch/1 -> Multiply/1
  Boolean signal/1 -> Switch/2
  Constant/1 -> Switch/3
  Constant1/1 -> Switch/1
  connections:
  Simulink-PS Converter2/RConn1 -- Control signal/RConn1

== system PandID/Valve Actuation Block1 ==
  Boolean signal : Inport
  Constant : Constant  Value=0
  Constant1 : Constant  Value=P_area
  Multiply : Gain  Gain=Valve_signal_Unit
  Simulink-PS Converter2 : nesl_utility/Simulink-PS Converter  PhysicalDomain=network_engine_domain  SubClassName=ps_input  LeftPortType=input  RightPortType=output  PseudoPeriodic=off  Frequencies=[]  NoiseDistribution=none  NoiseParameters=[]  Unit=m^2  AffineConversion=off  FilteringAndDerivatives=provide  SimscapeFilterOrder=1  InputFilterTimeConstant=0.001  UdotUserProvided=0
  Switch : Switch  Threshold=1
  Control signal : PMIOPort  Side=Right
  wires:
  Constant1/1 -> Switch/1
  Constant/1 -> Switch/3
  Boolean signal/1 -> Switch/2
  Switch/1 -> Multiply/1
  Multiply/1 -> Simulink-PS Converter2/1
  connections:
  Simulink-PS Converter2/RConn1 -- Control signal/RConn1

== system PandID/Valve Actuation Block10 ==
  Boolean signal : Inport
  Constant : Constant  Value=0
  Constant1 : Constant  Value=R_area
  Multiply : Gain  Gain=Valve_signal_Unit
  Simulink-PS Converter2 : nesl_utility/Simulink-PS Converter  PhysicalDomain=network_engine_domain  SubClassName=ps_input  LeftPortType=input  RightPortType=output  PseudoPeriodic=off  Frequencies=[]  NoiseDistribution=none  NoiseParameters=[]  Unit=m^2  AffineConversion=off  FilteringAndDerivatives=provide  SimscapeFilterOrder=1  InputFilterTimeConstant=0.001  UdotUserProvided=0
  Switch : Switch  Threshold=1
  Control signal : PMIOPort  Side=Right
  wires:
  Constant1/1 -> Switch/1
  Constant/1 -> Switch/3
  Boolean signal/1 -> Switch/2
  Switch/1 -> Multiply/1
  Multiply/1 -> Simulink-PS Converter2/1
  connections:
  Simulink-PS Converter2/RConn1 -- Control signal/RConn1

== system PandID/Valve Actuation Block11 ==
  Boolean signal : Inport
  Constant : Constant  Value=0
  Constant1 : Constant  Value=R_area
  Multiply : Gain  Gain=Valve_signal_Unit
  Simulink-PS Converter2 : nesl_utility/Simulink-PS Converter  PhysicalDomain=network_engine_domain  SubClassName=ps_input  LeftPortType=input  RightPortType=output  PseudoPeriodic=off  Frequencies=[]  NoiseDistribution=none  NoiseParameters=[]  Unit=m^2  AffineConversion=off  FilteringAndDerivatives=provide  SimscapeFilterOrder=1  InputFilterTimeConstant=0.001  UdotUserProvided=0
  Switch : Switch  Threshold=1
  Control signal : PMIOPort  Side=Right
  wires:
  Multiply/1 -> Simulink-PS Converter2/1
  Switch/1 -> Multiply/1
  Boolean signal/1 -> Switch/2
  Constant/1 -> Switch/3
  Constant1/1 -> Switch/1
  connections:
  Simulink-PS Converter2/RConn1 -- Control signal/RConn1

== system PandID/Valve Actuation Block2 ==
  Boolean signal : Inport
  Constant : Constant  Value=0
  Constant1 : Constant  Value=P_area
  Multiply : Gain  Gain=Valve_signal_Unit
  Simulink-PS Converter2 : nesl_utility/Simulink-PS Converter  PhysicalDomain=network_engine_domain  SubClassName=ps_input  LeftPortType=input  RightPortType=output  PseudoPeriodic=off  Frequencies=[]  NoiseDistribution=none  NoiseParameters=[]  Unit=m^2  AffineConversion=off  FilteringAndDerivatives=provide  SimscapeFilterOrder=1  InputFilterTimeConstant=0.001  UdotUserProvided=0
  Switch : Switch  Threshold=1
  Control signal : PMIOPort  Side=Right
  wires:
  Multiply/1 -> Simulink-PS Converter2/1
  Switch/1 -> Multiply/1
  Boolean signal/1 -> Switch/2
  Constant/1 -> Switch/3
  Constant1/1 -> Switch/1
  connections:
  Simulink-PS Converter2/RConn1 -- Control signal/RConn1

== system PandID/Valve Actuation Block3 ==
  Boolean signal : Inport
  Constant : Constant  Value=0
  Constant1 : Constant  Value=P_area
  Multiply : Gain  Gain=Valve_signal_Unit
  Simulink-PS Converter2 : nesl_utility/Simulink-PS Converter  PhysicalDomain=network_engine_domain  SubClassName=ps_input  LeftPortType=input  RightPortType=output  PseudoPeriodic=off  Frequencies=[]  NoiseDistribution=none  NoiseParameters=[]  Unit=m^2  AffineConversion=off  FilteringAndDerivatives=provide  SimscapeFilterOrder=1  InputFilterTimeConstant=0.001  UdotUserProvided=0
  Switch : Switch  Threshold=1
  Control signal : PMIOPort  Side=Right
  wires:
  Constant1/1 -> Switch/1
  Constant/1 -> Switch/3
  Boolean signal/1 -> Switch/2
  Switch/1 -> Multiply/1
  Multiply/1 -> Simulink-PS Converter2/1
  connections:
  Simulink-PS Converter2/RConn1 -- Control signal/RConn1

== system PandID/Valve Actuation Block4 ==
  Boolean signal : Inport
  Constant : Constant  Value=0
  Constant1 : Constant  Value=P_area
  Multiply : Gain  Gain=Valve_signal_Unit
  Simulink-PS Converter2 : nesl_utility/Simulink-PS Converter  PhysicalDomain=network_engine_domain  SubClassName=ps_input  LeftPortType=input  RightPortType=output  PseudoPeriodic=off  Frequencies=[]  NoiseDistribution=none  NoiseParameters=[]  Unit=m^2  AffineConversion=off  FilteringAndDerivatives=provide  SimscapeFilterOrder=1  InputFilterTimeConstant=0.001  UdotUserProvided=0
  Switch : Switch  Threshold=1
  Control signal : PMIOPort  Side=Right
  wires:
  Multiply/1 -> Simulink-PS Converter2/1
  Switch/1 -> Multiply/1
  Boolean signal/1 -> Switch/2
  Constant/1 -> Switch/3
  Constant1/1 -> Switch/1
  connections:
  Simulink-PS Converter2/RConn1 -- Control signal/RConn1

== system PandID/Valve Actuation Block5 ==
  Boolean signal : Inport
  Constant : Constant  Value=0
  Constant1 : Constant  Value=P_area
  Multiply : Gain  Gain=Valve_signal_Unit
  Simulink-PS Converter2 : nesl_utility/Simulink-PS Converter  PhysicalDomain=network_engine_domain  SubClassName=ps_input  LeftPortType=input  RightPortType=output  PseudoPeriodic=off  Frequencies=[]  NoiseDistribution=none  NoiseParameters=[]  Unit=m^2  AffineConversion=off  FilteringAndDerivatives=provide  SimscapeFilterOrder=1  InputFilterTimeConstant=0.001  UdotUserProvided=0
  Switch : Switch  Threshold=1
  Control signal : PMIOPort  Side=Right
  wires:
  Constant1/1 -> Switch/1
  Constant/1 -> Switch/3
  Boolean signal/1 -> Switch/2
  Switch/1 -> Multiply/1
  Multiply/1 -> Simulink-PS Converter2/1
  connections:
  Simulink-PS Converter2/RConn1 -- Control signal/RConn1

== system PandID/Valve Actuation Block6 ==
  Boolean signal : Inport
  Constant : Constant  Value=0
  Constant1 : Constant  Value=P_area
  Multiply : Gain  Gain=Valve_signal_Unit
  Simulink-PS Converter2 : nesl_utility/Simulink-PS Converter  PhysicalDomain=network_engine_domain  SubClassName=ps_input  LeftPortType=input  RightPortType=output  PseudoPeriodic=off  Frequencies=[]  NoiseDistribution=none  NoiseParameters=[]  Unit=m^2  AffineConversion=off  FilteringAndDerivatives=provide  SimscapeFilterOrder=1  InputFilterTimeConstant=0.001  UdotUserProvided=0
  Switch : Switch  Threshold=1
  Control signal : PMIOPort  Side=Right
  wires:
  Multiply/1 -> Simulink-PS Converter2/1
  Switch/1 -> Multiply/1
  Boolean signal/1 -> Switch/2
  Constant/1 -> Switch/3
  Constant1/1 -> Switch/1
  connections:
  Simulink-PS Converter2/RConn1 -- Control signal/RConn1

== system PandID/Valve Actuation Block7 ==
  Boolean signal : Inport
  Constant : Constant  Value=0
  Constant1 : Constant  Value=P_area
  Multiply : Gain  Gain=Valve_signal_Unit
  Simulink-PS Converter2 : nesl_utility/Simulink-PS Converter  PhysicalDomain=network_engine_domain  SubClassName=ps_input  LeftPortType=input  RightPortType=output  PseudoPeriodic=off  Frequencies=[]  NoiseDistribution=none  NoiseParameters=[]  Unit=m^2  AffineConversion=off  FilteringAndDerivatives=provide  SimscapeFilterOrder=1  InputFilterTimeConstant=0.001  UdotUserProvided=0
  Switch : Switch  Threshold=1
  Control signal : PMIOPort  Side=Right
  wires:
  Constant1/1 -> Switch/1
  Constant/1 -> Switch/3
  Boolean signal/1 -> Switch/2
  Switch/1 -> Multiply/1
  Multiply/1 -> Simulink-PS Converter2/1
  connections:
  Simulink-PS Converter2/RConn1 -- Control signal/RConn1

== system PandID/Valve Actuation Block8 ==
  Boolean signal : Inport
  Constant : Constant  Value=0
  Constant1 : Constant  Value=L_area
  Multiply : Gain  Gain=Valve_signal_Unit
  Simulink-PS Converter2 : nesl_utility/Simulink-PS Converter  PhysicalDomain=network_engine_domain  SubClassName=ps_input  LeftPortType=input  RightPortType=output  PseudoPeriodic=off  Frequencies=[]  NoiseDistribution=none  NoiseParameters=[]  Unit=m^2  AffineConversion=off  FilteringAndDerivatives=provide  SimscapeFilterOrder=1  InputFilterTimeConstant=0.001  UdotUserProvided=0
  Switch : Switch  Threshold=1
  Control signal : PMIOPort  Side=Right
  wires:
  Multiply/1 -> Simulink-PS Converter2/1
  Switch/1 -> Multiply/1
  Boolean signal/1 -> Switch/2
  Constant/1 -> Switch/3
  Constant1/1 -> Switch/1
  connections:
  Simulink-PS Converter2/RConn1 -- Control signal/RConn1

== system PandID/Valve Actuation Block9 ==
  Boolean signal : Inport
  Constant : Constant  Value=0
  Constant1 : Constant  Value=L_area
  Multiply : Gain  Gain=Valve_signal_Unit
  Simulink-PS Converter2 : nesl_utility/Simulink-PS Converter  PhysicalDomain=network_engine_domain  SubClassName=ps_input  LeftPortType=input  RightPortType=output  PseudoPeriodic=off  Frequencies=[]  NoiseDistribution=none  NoiseParameters=[]  Unit=m^2  AffineConversion=off  FilteringAndDerivatives=provide  SimscapeFilterOrder=1  InputFilterTimeConstant=0.001  UdotUserProvided=0
  Switch : Switch  Threshold=1
  Control signal : PMIOPort  Side=Right
  wires:
  Constant1/1 -> Switch/1
  Constant/1 -> Switch/3
  Boolean signal/1 -> Switch/2
  Switch/1 -> Multiply/1
  Multiply/1 -> Simulink-PS Converter2/1
  connections:
  Simulink-PS Converter2/RConn1 -- Control signal/RConn1
